simulink model "untitled22"  (R2019b)
settings: Solver=FixedStepAuto  StartTime=0.0  StopTime=50  FixedStep=1e-3  RelTol=1e-3
values from neighbouring files (symbols this model uses):
  B = 0.1    [uloha3.m]
  b = 0.05    [uloha3.m]
  Kv = -1/g    (= -0.101936799185)    [uloha3.m]
  l = 3    [uloha3.m]
  omega = sqrt(g/l)    [uloha3.m]
  Tm = 1    [uloha3.m]
undefined symbols (not defined in the file or in its folder): A, jerk, sigbuilder_block
libraries: vrlib x3
settings Model: Creator=Niki  LastModifiedBy=Niki

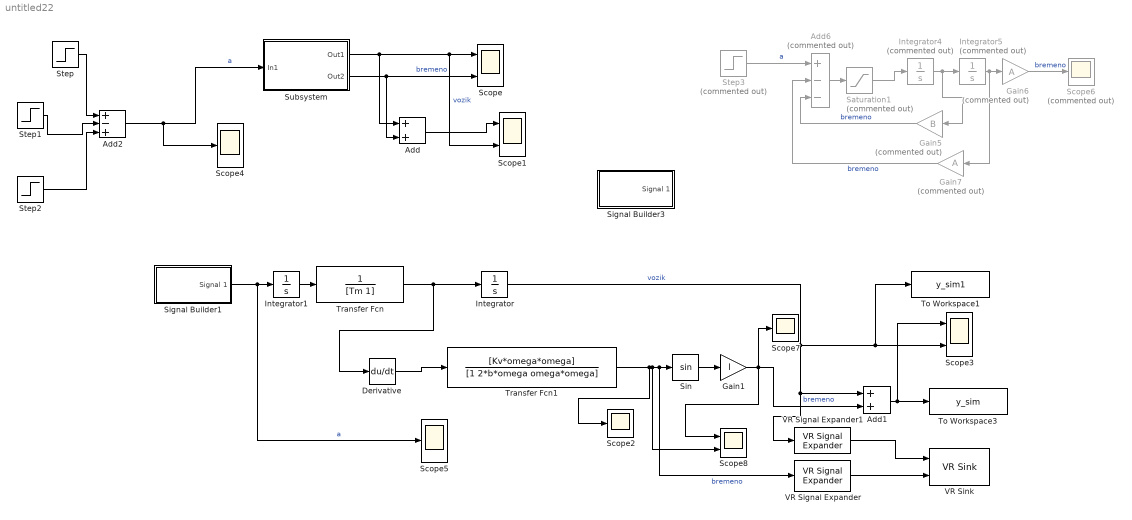
== system untitled22 ==
  Add : Sum
  Add1 : Sum
  Add2 : Sum  Inputs=+-+
  Add6 : Sum  Commented=on  Inputs=+--
  Derivative : Derivative
  Gain1 : Gain  Gain=l
  Gain5 : Gain  Commented=on  Gain=B
  Gain6 : Gain  Commented=on  Gain=A
  Gain7 : Gain  Commented=on  Gain=A
  Integrator : Integrator
  Integrator1 : Integrator
  Integrator4 : Integrator  Commented=on
  Integrator5 : Integrator  Commented=on
  Saturation1 : Saturate  Commented=on  UpperLimit=jerk  LowerLimit=-jerk
  Scope{,1,3,8} (4 alike) : Scope  NumInputPorts=2
  Scope{2,4..5,7} (4 alike) : Scope
  Scope6 : Scope  Commented=on
  Signal Builder1 : Subsystem  Tag=STV Subsys  LoadFcn=sigbuilder_block('load');  StartFcn=sigbuilder_block('start');  StopFcn=sigbuilder_block('stop');  ClipboardFcn=sigbuilder_block('clipboard');  mask(Sigbuilder block){tuvar=[0:10]}
      mask help: Simulink:masks:SigbuilderBlock_MD
      mask init:
      | if ~strcmp(get_param(bdroot(gcbh),'SimulationStatus'),'stopped') tuvar = sigbuilder_block('maskInit'); end
      settings: CopyFcn=sigbuilder_block('copy');  DeleteFcn=sigbuilder_block('delete');  ModelCloseFcn=sigbuilder_block('modelClose');  PreSaveFcn=sigbuilder_block('preSave');  PauseFcn=sigbuilder_block('pause');  ContinueFcn=sigbuilder_block('continue');  NameChangeFcn=sigbuilder_block('namechange');  OpenFcn=sigbuilder_block('open',[136.2 112.2 550.8 400.2 ]);  CloseFcn=sigbuilder_block('close');
      mask Display: plot(0, 0, 100, 100,[2, 2, 32, 32, 2], [68, 8, 8, 68, 68],[32, 2], [38, 38], [32, 19, 2],[53, 60, 44], [32, 17, 17, 2],[16, 16, 31, 31]);txt = getActiveGroup(gcbh);text(2, 100, txt,'verticalAlignment', 'top');
  Signal Builder3 : Subsystem  Tag=STV Subsys  LoadFcn=sigbuilder_block('load');  StartFcn=sigbuilder_block('start');  StopFcn=sigbuilder_block('stop');  ClipboardFcn=sigbuilder_block('clipboard');  mask(Sigbuilder block){tuvar=[0:10]}
      mask help: Simulink:masks:SigbuilderBlock_MD
      mask init:
      | if ~strcmp(get_param(bdroot(gcbh),'SimulationStatus'),'stopped') tuvar = sigbuilder_block('maskInit'); end
      settings: CopyFcn=sigbuilder_block('copy');  DeleteFcn=sigbuilder_block('delete');  ModelCloseFcn=sigbuilder_block('modelClose');  PreSaveFcn=sigbuilder_block('preSave');  PauseFcn=sigbuilder_block('pause');  ContinueFcn=sigbuilder_block('continue');  NameChangeFcn=sigbuilder_block('namechange');  OpenFcn=sigbuilder_block('open',[136.2 112.2 550.8 400.2 ]);  CloseFcn=sigbuilder_block('close');
      mask Display: plot(0, 0, 100, 100,[2, 2, 32, 32, 2], [68, 8, 8, 68, 68],[32, 2], [38, 38], [32, 19, 2],[53, 60, 44], [32, 17, 17, 2],[16, 16, 31, 31]);txt = getActiveGroup(gcbh);text(2, 100, txt,'verticalAlignment', 'top');
  Sin : Trigonometry
  Step : Step  SampleTime=0
  Step1 : Step  Time=2  After=2  SampleTime=0
  Step2 : Step  Time=3  SampleTime=0
  Step3 : Step  Commented=on  SampleTime=0
  Subsystem : Subsystem
  To Workspace1 : ToWorkspace  VariableName=y_sim1  SaveFormat=Timeseries  SampleTime=-1
  To Workspace3 : ToWorkspace  VariableName=y_sim  SaveFormat=Timeseries  SampleTime=-1
  Transfer Fcn : TransferFcn  Denominator=[Tm 1]
  Transfer Fcn1 : TransferFcn  Numerator=[Kv*omega*omega]  Denominator=[1 2*b*omega omega*omega]
  VR Signal Expander : vrlib/VR Signal Expander  outwidth=4  outidx=[4]
      settings: SourceProductName=Simulink
  VR Signal Expander1 : vrlib/VR Signal Expander  outwidth=3  outidx=1
      settings: SourceProductName=Simulink
  VR Sink : vrlib/VR Sink  InstantiateOnLoad=on  SampleTime=0.1  ViewEnable=on  RemoteChange=off  RemoteView=off  FieldsWritten=Car.translation.3.1.1.double#klb.rotation.4.1.1.double  WorldFileName=vrml1.wrl  AutoView=off  VideoDimensions=[]  AllowVariableSize=off
      settings: SourceProductName=Simulink
  wires:
  Subsystem/2(Out2) -> Add/2, Scope/2  "bremeno"
  Subsystem/1(Out1) -> Add/1, Scope1/2, Scope/1  "vozik"
  Step1/1 -> Add2/2
  Step2/1 -> Add2/3
  Step/1 -> Add2/1
  Add2/1 -> Scope4/1, Subsystem/1(In1)  "a"
  Add/1 -> Scope1/1
  Signal Builder1/1(Signal 1) -> Scope5/1, Integrator1/1  "a"
  Sin/1 -> Gain1/1
  Integrator1/1 -> Transfer Fcn/1
  Transfer Fcn1/1 -> Scope2/1, Scope8/2, VR Signal Expander/1, Sin/1  "bremeno"
  Add1/1 -> To Workspace3/1, Scope3/1
  Derivative/1 -> Transfer Fcn1/1
  Transfer Fcn/1 -> Derivative/1, Integrator/1
  Integrator/1 -> To Workspace1/1, Scope3/2, Add1/1, VR Signal Expander1/1  "vozik"
  Gain1/1 -> Scope8/1, Scope7/1, Add1/2  "bremeno"
  Saturation1/1 -> Integrator4/1
  Gain6/1 -> Scope6/1  "bremeno"
  Gain7/1 -> Add6/2  "bremeno"
  Add6/1 -> Saturation1/1
  Step3/1 -> Add6/1  "a"
  Gain5/1 -> Add6/3  "bremeno"
  Integrator4/1 -> Integrator5/1, Gain5/1
  Integrator5/1 -> Gain6/1, Gain7/1
  VR Signal Expander/1 -> VR Sink/2
  VR Signal Expander1/1 -> VR Sink/1

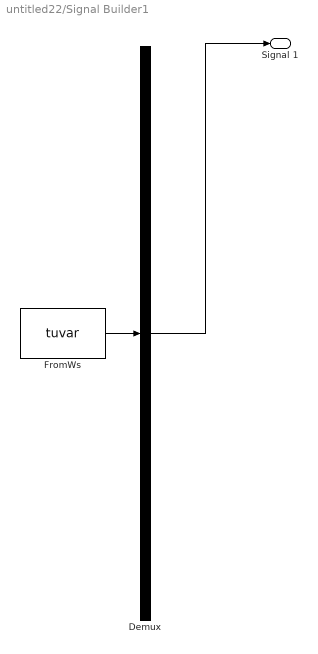
== system untitled22/Signal Builder1 ==
  Demux : Demux  Tag=STV Demux  Outputs=1
  FromWs : FromWorkspace  Tag=STV FromWs  VariableName=tuvar  SampleTime=0
      SigBuilderData=|
      | common.afterFinalStr = 'Extrapolate'
      | common.sampleTime = 0
      | dataSet.timeRange = [0 10]
      | dataSet.name = 'Group 1'
      | sbobj.Groups.Name = 'Group 1'
      | sbobj.Groups.Signals.Name = 'Signal 1'
      | sbobj.Groups.Signals.XData = [0 1 1 2 2 3 3 10]
      | sbobj.Groups.Signals.YData = [0 0 10 10 -10 -10 0 0]
  Signal 1 : Outport  Tag=STV Outport
  wires:
  FromWs/1 -> Demux/1
  Demux/1 -> Signal 1/1

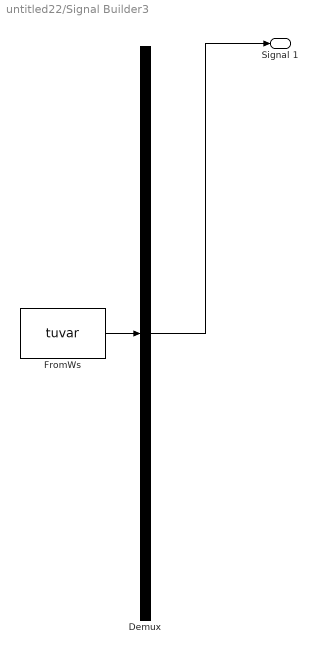
== system untitled22/Signal Builder3 ==
  Demux : Demux  Tag=STV Demux  Outputs=1
  FromWs : FromWorkspace  Tag=STV FromWs  VariableName=tuvar  SampleTime=0
      SigBuilderData=|
      | common.afterFinalStr = 'Extrapolate'
      | common.sampleTime = 0
      | dataSet.timeRange = [0 10]
      | dataSet.name = 'Group 1'
      | sbobj.Groups.Name = 'Group 1'
      | sbobj.Groups.Signals.Name = 'Signal 1'
      | sbobj.Groups.Signals.XData = [0 1 1 2 2 3 3 10]
      | sbobj.Groups.Signals.YData = [0 0 1 1 -1 -1 0 0]
  Signal 1 : Outport  Tag=STV Outport
  wires:
  FromWs/1 -> Demux/1
  Demux/1 -> Signal 1/1

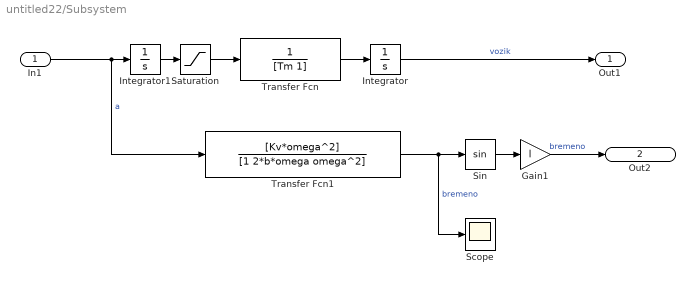
== system untitled22/Subsystem ==
  In1 : Inport
  Gain1 : Gain  Gain=l
  Integrator : Integrator
  Integrator1 : Integrator
  Saturation : Saturate  UpperLimit=20  LowerLimit=-20
  Scope : Scope
  Sin : Trigonometry
  Transfer Fcn : TransferFcn  Denominator=[Tm 1]
  Transfer Fcn1 : TransferFcn  Numerator=[Kv*omega^2]  Denominator=[1 2*b*omega omega^2]
  Out1 : Outport
  Out2 : Outport  Port=2
  wires:
  In1/1 -> Transfer Fcn1/1, Integrator1/1  "a"
  Integrator/1 -> Out1/1  "vozik"
  Integrator1/1 -> Saturation/1
  Transfer Fcn/1 -> Integrator/1
  Transfer Fcn1/1 -> Scope/1, Sin/1  "bremeno"
  Sin/1 -> Gain1/1
  Saturation/1 -> Transfer Fcn/1
  Gain1/1 -> Out2/1  "bremeno"
